simulink model "commdvbs2"  (R2017a)
settings: Solver=FixedStepDiscrete  StartTime=0.0  StopTime=10  RelTol=1e-3
PostLoadFcn:
  | commdvbs2_settings;
undefined symbols (not defined in the file or in its folder): dvb
libraries: commblkcod2 x4, dspsigops x2, commsink2 x2, commblkintrlv2 x2, commdigbbndpm3 x2, dspstat3 x2, commchan3 x1, dspobslib x1, commblksprivate x1, commrandsrc3 x1, dspmathops x1
Description:
  | DVB-S.2 Link, Including LDPC Coding
settings Model: ExtModeAutoUpdateStatusClock=off  Creator=The MathWorks, Inc.  LastModifiedBy=ikhaliqu
settings SolverCC: InsertRTBMode=Auto
settings DataIOCC: LimitDataPoints=on  SaveFormat=Array  SaveOutput=off  SignalLogging=off  SaveTime=off
settings OptimizationCC: DefaultParameterBehavior=Inlined  ExpressionDepthLimit=2147483647  RollThreshold=2  InitFltsAndDblsToZero=on  EfficientMapNaN2IntZero=off  LifeSpan=inf
settings DebuggingCC: AlgebraicLoopMsg=error  UnderspecifiedInitializationDetection=Classic  MergeDetectMultiDrivingBlocksExec=none  SignalResolutionControl=TryResolveAllWithWarning  SolverPrmCheckMsg=warning  MultiTaskDSMMsg=warning  MultiTaskCondExecSysMsg=none  SingleTaskRateTransMsg=error  FcnCallInpInsideContextMsg=warning  AllowSymbolicDim=off  StateNameClashWarn=warning  SFUnexpectedBacktrackingDiag=warning  SFNoUnconditionalDefaultTransitionDiag=warning  SFExecutionAtInitializationDiag=none
settings HardwareCC: ProdBitPerPointer=32  ProdBitPerSizeT=32  ProdBitPerPtrDiffT=32  ProdLargestAtomicFloat=None  ProdIntDivRoundTo=Undefined  ProdEndianess=Unspecified  ProdWordSize=32  ProdHWDeviceType=32-bit Generic
settings ModelReferenceCC: PropagateSignalLabelsOutOfModel=off
settings SFSimCC: SFSimEcho=off  SimParseCustomCode=off
settings RTWCC: GenerateReport=on  LaunchReport=on
settings GRTTargetCC: TargetFcnLib=ansi_tfl_tmw_new.mat  TargetLangStandard=C89/C90 (ANSI)  GeneratePreprocessorConditionals=Disable all  CombineOutputUpdateFcns=off  GRTInterface=on
settings ConfigComp: CovMetricSettings=dw  CovHtmlReporting=on  CovSaveCumulativeToWorkspaceVar=on  CovSaveSingleToWorkspaceVar=on  CovExternalEMLEnable=off  CovSFcnEnable=off

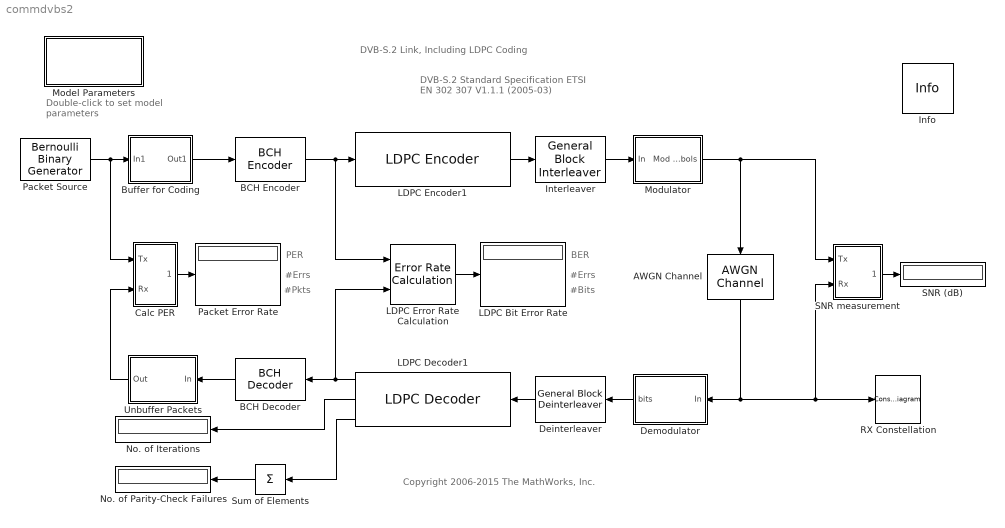
== system commdvbs2 ==
  note: DVB-S.2 Link, Including LDPC Coding
  note: Double-click to
      | set model parameters
  note: DVB-S.2 Standard Specification
      | ETSI EN 302 307 V1.1.1 (2005-03)
  note: PER
  note: #Pkts
  note: #Errs
  note: BER
  note: #Bits
  note: #Errs
  note: Copyright 2006-2015 The MathWorks, Inc.
  AWGN Channel : commchan3/AWGN Channel  InputProcessing=Columns as channels (frame based)  seed=dvb.seed  noiseMode=Variance from mask  EbNodB=10  EsNodB=10  SNRdB=10  bitsPerSym=1  Ps=1  Tsym=1  variance=dvb.NoiseVar
  BCH Decoder : commblkcod2/BCH Decoder  n=dvb.BCHCodewordLength  k=dvb.BCHMessageLength  specShortening=off  shortenedK=5  specGenPoly=on  genPoly=dvb.BCHGeneratorPoly  specPrimPoly=on  prPoly=dvb.BCHPrimitivePoly  specDisableGenCheck=on  specPuncture=off  punctVec=[ones(8,1); zeros(2,1)]  specErasurePort=off  showNumErr=off
      settings: SourceProductName=Communications System Toolbox  SourceProductBaseCode=CM
  BCH Encoder : commblkcod2/BCH Encoder  n=dvb.BCHCodewordLength  k=dvb.BCHMessageLength  specShortening=off  shortenedK=5  specGenPoly=on  genPoly=dvb.BCHGeneratorPoly  specPrimPoly=on  prPoly=dvb.BCHPrimitivePoly  specDisableGenCheck=on  specPuncture=off  punctVec=[ones(8,1); zeros(2,1)]
      settings: SourceProductName=Communications System Toolbox  SourceProductBaseCode=CM
  Buffer for Coding : Subsystem
      mask Display: disp('BBFRAME\nBuffering')
  Calc PER : Subsystem
  Deinterleaver : commblkintrlv2/General Block Deinterleaver  permutationVectorSource=Dialog  elements=dvb.InterleaveOrder
      settings: SourceProductName=Communications System Toolbox  SourceProductBaseCode=CM
  Demodulator : Subsystem
      mask init:
      | dvb = evalin('base', 'dvb');
      mask Display: disp([dvb.ModulationType '\nSoft-Decision\nDemodulator'])
  Info : commblksprivate/Info  SystemSampleTime=-1
      settings: SourceProductName=Communications System Toolbox  SourceProductBaseCode=CM
  Interleaver : commblkintrlv2/General Block Interleaver  permutationVectorSource=Dialog  elements=dvb.InterleaveOrder
      settings: SourceProductName=Communications System Toolbox  SourceProductBaseCode=CM
  LDPC Bit Error Rate : Display
  LDPC Decoder1 : commblkcod2/LDPC Decoder  ParityCheckMat=dvb.LDPCParityCheckMatrix  OutputFmt=Information part  DecisionType=Hard decision  OutputDataType=boolean  NumIter=dvb.LDPCNumIterations  DoParityCheck=on  OutputNumIter=on  OutputFinalChecks=on
      settings: SourceProductName=Communications System Toolbox  SourceProductBaseCode=CM
  LDPC Encoder1 : commblkcod2/LDPC Encoder  ParityCheckMat=dvb.LDPCParityCheckMatrix
      settings: SourceProductName=Communications System Toolbox  SourceProductBaseCode=CM
  LDPC Error Rate Calculation : commsink2/Error Rate Calculation  N=0  st_delay=dvb.BCHCodewordLength  cp_mode=Entire frame  subframe=[]  PMode=Port  WsName=ErrorVec  RsMode2=off  stop=off  numErr=100  maxBits=1e6
  Model Parameters : Subsystem  mask(Model Parameters){modulationAndCodingMode=QPSK 3/4, EsNodB=20, LDPCNumIterations=50, seed=25}
      mask prompts: modulationAndCodingMode "Mode:"; EsNodB "Es/No (dB):"; LDPCNumIterations "Number of iterations for LDPC decoder:"; seed "Seed (for random data and noise):"
      mask help: Specifies model parameters.
      mask init:
      | commdvbs2_settings;
      mask Help: helpview(commdhelp);
      mask TypeOptions modulationAndCodingMode: QPSK 1/4 | QPSK 1/3 | QPSK 2/5 | QPSK 1/2 | QPSK 3/5 | QPSK 2/3 | QPSK 3/4 | QPSK 4/5 | QPSK 5/6 | QPSK 8/9 | QPSK 9/10 | 8PSK 3/5 | 8PSK 2/3 | 8PSK 3/4 | 8PSK 5/6 | 8PSK 8/9 | 8PSK 9/10
      mask Display: disp('Model\nParameters')
  Modulator : Subsystem
      mask init:
      | dvb = evalin('base', 'dvb');
      mask Display: disp([dvb.ModulationType '\nModulator' ])
  No. of Iterations : Display
  No. of Parity-Check Failures : Display
  Packet Error Rate : Display
  Packet Source : commrandsrc3/Bernoulli Binary Generator  ProbabilityOfZero=0.5  SeedSource=Parameter  Seed=dvb.seed  SampleTime=dvb.BitPeriod  SamplesPerFrame=dvb.NumBitsPerPacket  OutputDataType=boolean  SimulateUsing=Interpreted execution
  RX Constellation : ConstellationDiagram  Tag=ScatterPlot
  SNR measurement : Subsystem
  SNR (dB) : Display
  Sum of Elements : Sum  Inputs=+
  Unbuffer Packets : Subsystem
      mask Display: disp('BBFRAME\nUnbuffering')
  wires:
  LDPC Error Rate Calculation/1 -> LDPC Bit Error Rate/1
  BCH Encoder/1 -> LDPC Error Rate Calculation/1, LDPC Encoder1/1
  Interleaver/1 -> Modulator/1(In)
  Modulator/1(Mod Symbols) -> SNR measurement/1(Tx), AWGN Channel/1
  Packet Source/1 -> Calc PER/1(Tx), Buffer for Coding/1(In1)
  Buffer for Coding/1(Out1) -> BCH Encoder/1
  Demodulator/1(bits) -> Deinterleaver/1
  SNR measurement/1(SNRdB) -> SNR (dB)/1
  AWGN Channel/1 -> SNR measurement/2(Rx), RX Constellation/1, Demodulator/1(In)
  Calc PER/1(PER) -> Packet Error Rate/1
  Unbuffer Packets/1(Out) -> Calc PER/2(Rx)
  BCH Decoder/1 -> Unbuffer Packets/1(In)
  LDPC Encoder1/1 -> Interleaver/1
  LDPC Decoder1/1 -> LDPC Error Rate Calculation/2, BCH Decoder/1
  Sum of Elements/1 -> No. of Parity-Check Failures/1
  Deinterleaver/1 -> LDPC Decoder1/1
  LDPC Decoder1/3 -> Sum of Elements/1
  LDPC Decoder1/2 -> No. of Iterations/1

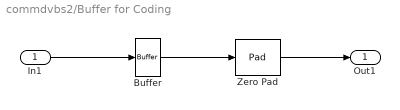
== system commdvbs2/Buffer for Coding ==
  In1 : Inport
  Buffer : Buffer  N=dvb.NumInfoBitsPerCodeword  OutputFrames=off
  Zero Pad : dspsigops/Pad  padAlong=Columns  dimsToPad=1  valSrc=Specify via dialog  padVal=0  spec=Output size  padNumOutRowsSpecMethod=User-specified  numOutRows=dvb.BCHMessageLength  padNumOutColsSpecMethod=User-specified  numOutCols=1  isVarDimsMode=off  padBeginning=0  padEnd=0  outSizeMode=User-specified  outSize=1  padSigAt=End  trunc_flag=None  roundingMode=Floor  overflowMode=off  truncOrWrapMode=Truncate  wrap_flag=None
      settings: SourceProductName=DSP System Toolbox  SourceProductBaseCode=DS
  Out1 : Outport
  wires:
  In1/1 -> Buffer/1
  Buffer/1 -> Zero Pad/1
  Zero Pad/1 -> Out1/1

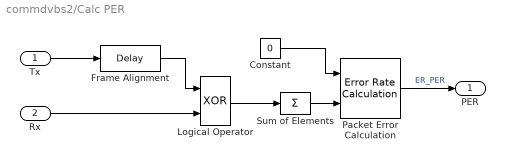
== system commdvbs2/Calc PER ==
  Tx : Inport
  Rx : Inport  Port=2
  Constant : Constant  Value=0  OutDataTypeStr=double
  Frame Alignment : dspobslib/Delay  InputProcessing=Columns as channels (frame based)  dly_unit=Samples  delay=dvb.NumInfoBitsPerCodeword  ic_detail=off  dif_ic_for_ch=off  dif_ic_for_dly=off  ic=0  reset_popup=None
      settings: SourceProductName=DSP System Toolbox  SourceProductBaseCode=DS
  Logical Operator : Logic  Operator=XOR  AllPortsSameDT=off  OutDataTypeStr=boolean
  Packet Error Calculation : commsink2/Error Rate Calculation  N=0  st_delay=dvb.NumInfoBitsPerCodeword/dvb.NumBitsPerPacket  cp_mode=Entire frame  subframe=[]  PMode=Port  WsName=ErrorVec  RsMode2=off  stop=off  numErr=100  maxBits=1e6
  Sum of Elements : Sum  Inputs=+  OutDataTypeStr=double
  PER : Outport
  wires:
  Constant/1 -> Packet Error Calculation/1
  Rx/1 -> Logical Operator/2
  Packet Error Calculation/1 -> PER/1  "ER_PER"
  Tx/1 -> Frame Alignment/1
  Frame Alignment/1 -> Logical Operator/1
  Logical Operator/1 -> Sum of Elements/1
  Sum of Elements/1 -> Packet Error Calculation/2

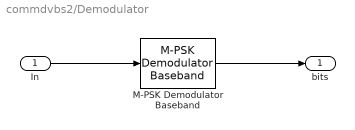
== system commdvbs2/Demodulator ==
  In : Inport
  M-PSK Demodulator Baseband : commdigbbndpm3/M-PSK Demodulator Baseband  M=2^dvb.BitsPerSymbol  OutType=Bit  DecType=Approximate log-likelihood ratio  VarSource=Dialog  Variance=dvb.NoiseVar  Dec=User-defined  Mapping=dvb.SymbolMapping  Ph=dvb.PhaseOffset  outDtype1=double  outDtype2=double  derotateFactorWordLen=16  derotateFactorDataTypeStr=Inherit: Same word length as input  derotateFactorLastDataTypeStr=Inherit: Same word length as input
      settings: SourceProductName=Communications System Toolbox
  bits : Outport
  wires:
  In/1 -> M-PSK Demodulator Baseband/1
  M-PSK Demodulator Baseband/1 -> bits/1

== system commdvbs2/Model Parameters ==
  note: This subsystem is empty.
      | It is used for setting parameter values (in the mask).

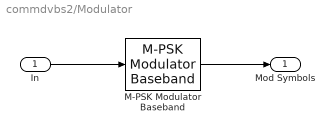
== system commdvbs2/Modulator ==
  In : Inport
  M-PSK Modulator Baseband : commdigbbndpm3/M-PSK Modulator Baseband  M=2^dvb.BitsPerSymbol  InType=Bit  Enc=User-defined  Mapping=dvb.SymbolMapping  Ph=dvb.PhaseOffset  outDtype=double  outWordLen=16  outUDDataType=sfix(16)  outFracLenMode=Best precision  outFracLen=15  outDataTypeStr=double  outLastDataTypeStr=double
      settings: SourceProductName=Communications System Toolbox
  Mod Symbols : Outport
  wires:
  In/1 -> M-PSK Modulator Baseband/1
  M-PSK Modulator Baseband/1 -> Mod Symbols/1

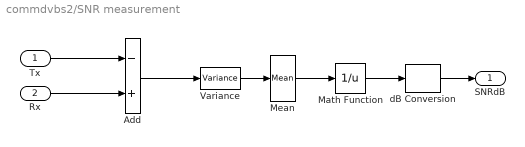
== system commdvbs2/SNR measurement ==
  Tx : Inport
  Rx : Inport  Port=2
  Add : Sum  Inputs=-+
  Math Function : Math  Operator=reciprocal  SaturateOnIntegerOverflow=on
  Mean : dspstat3/Mean  run=off  reset_popup=Non-zero sample  InputProcessing=Columns as channels (frame based)  directionMode=Each column  dimension=1  roiEnable=off  roiType=Rectangles  roiPortion=Entire ROI  roiOutput=Individual statistics for each ROI  roiFlag=off  outputDataTypeStr=Inherit: Same as accumulator  outputLastDataTypeStr=Inherit: Same as accumulator  outputMin=[]  outputMax=[]  roundingMode=Floor  overflowMode=off
  Variance : dspstat3/Variance  run=off  reset_popup=None  InputProcessing=Columns as channels (frame based)  directionMode=Each column  dimension=1  roiEnable=off  roiType=Rectangles  roiPortion=Entire ROI  roiOutput=Individual statistics for each ROI  roiFlag=off  roundingMode=Floor  overflowMode=off
      settings: SourceProductName=DSP System Toolbox
  dB Conversion : dspmathops/dB Conversion  dBtype=dB  intype=Power  R=1  fuzz=off
      settings: SourceProductName=DSP System Toolbox
  SNRdB : Outport
  wires:
  Add/1 -> Variance/1
  Variance/1 -> Mean/1
  Math Function/1 -> dB Conversion/1
  Mean/1 -> Math Function/1
  Tx/1 -> Add/1
  dB Conversion/1 -> SNRdB/1
  Rx/1 -> Add/2

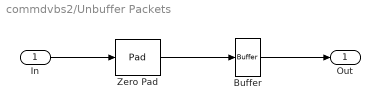
== system commdvbs2/Unbuffer Packets ==
  In : Inport
  Buffer : Buffer  N=dvb.NumBitsPerPacket  OutputFrames=off
  Zero Pad : dspsigops/Pad  padAlong=Columns  dimsToPad=1  valSrc=Specify via dialog  padVal=0  spec=Output size  padNumOutRowsSpecMethod=User-specified  numOutRows=dvb.NumInfoBitsPerCodeword  padNumOutColsSpecMethod=User-specified  numOutCols=1  isVarDimsMode=off  padBeginning=0  padEnd=0  outSizeMode=User-specified  outSize=1  padSigAt=End  trunc_flag=None  roundingMode=Floor  overflowMode=off  truncOrWrapMode=Truncate  wrap_flag=None
      settings: SourceProductName=DSP System Toolbox  SourceProductBaseCode=DS
  Out : Outport
  wires:
  In/1 -> Zero Pad/1
  Zero Pad/1 -> Buffer/1
  Buffer/1 -> Out/1
